simulink model "uz_mpc_6ph_sca"  (R2022b)
settings: Solver=FixedStepDiscrete  StartTime=0.0  StopTime=ST  RelTol=1e-3
InitFcn:
  | clear
  | clc
  | 
  | f_clock = 100e6;        % IP core clock freq in Hz
  | t_clock = 1/f_clock;    % IP core sample time in s
  | 
  | f_ADC =100e3;           % ADC interrupt freq in Hz
  | t_ADC = 1/f_ADC;        % ADC sample time in s
  | Ts = t_ADC;
  | 
  | % amplitude of sinusoidal signal sources
  | A = 0.1;
  | 
  | % machine parameters
  | Rs = 0.27;              % Phase resistance in Ohm
  | psi_pm = 0.19;          % PM flux linkage in Vs
  | Ld = 1.7e-3;            % d-inductance in H
  | Lq = 3.8e-3;            % q-inductance in H
  | Lx = 2.4e-3;            % x-inductance in H
  | Ly = 2.5e-3;            % y-inductance in H
  | p = 5;                  % pole pairs
  | 
  | VR = 400;               % Rated eff. line-line voltage in V
  | IR = 10/sqrt(2);             % Rated eff. phase current in A
  | % IR = 14.142;
  | nR = 3000;              % Rated mechanical speed in 1/min
  | 
  | % p.u. base units acc. to T.Geyer, Model predictive control of high power
  | % converters and industrial drives. Hoboken, NJ, USA: Wiley, 2016, Chapter 2.1.2
  | VB = sqrt(2/3)*VR;
  | IB = sqrt(2)*IR;
  | omegaB = nR*2*pi()/60*p;
  | ZB = VB/IB;
  | LB = ZB/omegaB;
  | SB = 3/2 *VB*IB;
  | psiB = VB/omegaB;
  | TB = psiB*IB;
  | 
  | %pre calculated constants - check results regarding fixd_type_constants!!!
  | Rs_over_ZB = Rs/ZB;
  | Ts_times_ZB_over_Ld = Ts*ZB/Ld;
  | Ts_times_ZB_over_Lq = Ts*ZB/Lq;
  | Ts_times_ZB_over_Lx = Ts*ZB/Lx;
  | Ts_times_ZB_over_Ly = Ts*ZB/Ly;
  | Ld_over_LB = Ld/LB;
  | Lq_over_LB = Lq/LB;
  | Ld_minus_Lq_over_LB = (Ld-Lq)/LB;
  | psi_pm_over_psiB = psi_pm/psiB;
  | 
  | % fixed-point data types
  | pu_fixdt_type = fixdt(1,18,15); % output data type of pu values
  | % fixdt_type_dq_currents = fixdt(1,27,16);
  | fixdt_type_dq_currents = fixdt(1,27,24);
  | fixdt_type_xy_currents = fixdt(1,18,11);
  | fixdt_type_dqxy_ref_currents = fixdt(1,18,15);
  | fixdt_type_dqxy_voltages = fixdt(1,27,24);
  | fixdt_type_angle = fixdt(1,24,20);
  | % fixdt_type_sin_cos = fixdt(1,18,16);
  | fixdt_type_sin_cos = fixdt(1,27,20);
  | fixdt_type_lambda = fixdt(0,18,17);
  | ... (+38 lines)
libraries: nesl_utility x44, fl_lib x41, simulink x23, ee_lib x12, hdlsllib x2, spsAlphaBetaZerotodq0Lib x1, batteryecm_lib x1
(part 3 of 4)

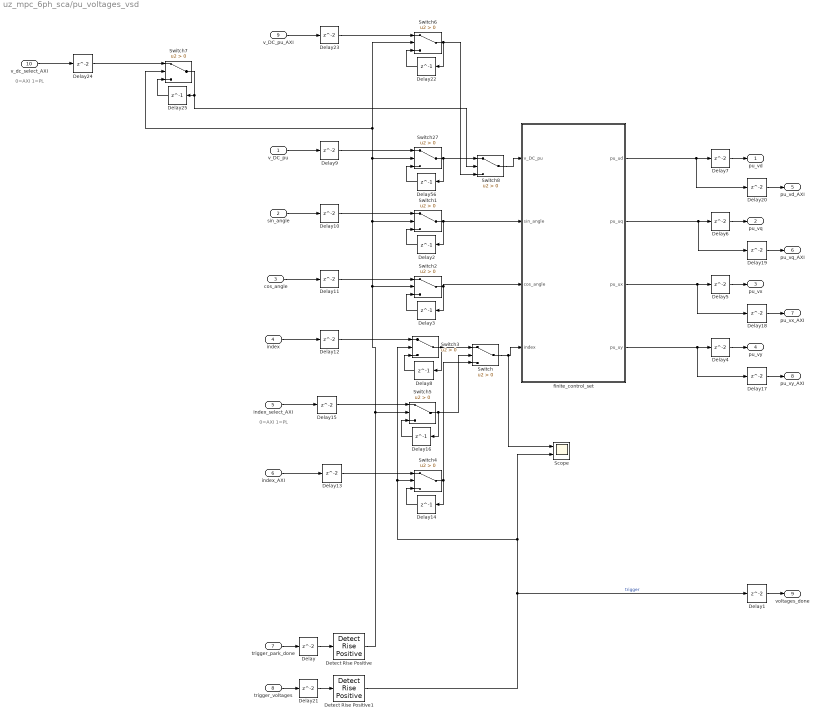
== system uz_mpc_6ph_sca/pu_voltages_vsd ==
  note: 0=AXI 1=PL
  note: 0=AXI 1=PL
  v_DC_pu : Inport  OutDataTypeStr=fixdt_type_constants
  sin_angle : Inport  Port=2  OutDataTypeStr=fixdt_type_sin_cos
  cos_angle : Inport  Port=3  OutDataTypeStr=fixdt_type_sin_cos
  index : Inport  Port=4
  index_select_AXI : Inport  Port=5
  index_AXI : Inport  Port=6
  trigger_park_done : Inport  Port=7
  trigger_voltages : Inport  Port=8
  v_DC_pu_AXI : Inport  Port=9  OutDataTypeStr=fixdt_type_constants
  v_dc_select_AXI : Inport  Port=10
  Delay{,1,4..7,9..11,17..21,23} (15 alike) : Delay
  Delay{12..13,15,24} (4 alike) : Delay  InitialCondition=1
  Delay{8,14,16,25} (4 alike) : Delay  DelayLength=1  InitialCondition=1
  Delay{2..3,22,56} (4 alike) : Delay  DelayLength=1
  Detect Rise Positive : simulink/Logic and Bit Operations/Detect Rise Positive  vinit=0  OutDataTypeStr=boolean
  Detect Rise Positive1 : simulink/Logic and Bit Operations/Detect Rise Positive  vinit=0  OutDataTypeStr=boolean
  Scope : Scope  NumInputPorts=2
  Switch : Switch  Criteria=u2 > Threshold  SaturateOnIntegerOverflow=off  InputSameDT=off
  Switch1 : Switch  Criteria=u2 > Threshold  OutDataTypeStr=fixdt_type_sin_cos  SaturateOnIntegerOverflow=off  InputSameDT=off
  Switch2 : Switch  Criteria=u2 > Threshold  OutDataTypeStr=fixdt_type_sin_cos  SaturateOnIntegerOverflow=off  InputSameDT=off
  Switch27 : Switch  Criteria=u2 > Threshold  OutDataTypeStr=fixdt_type_constants  SaturateOnIntegerOverflow=off  InputSameDT=off
  Switch{3..5,7} (4 alike) : Switch  Criteria=u2 > Threshold  OutDataTypeStr=fixdt_type_polepairs  SaturateOnIntegerOverflow=off  InputSameDT=off
  Switch6 : Switch  Criteria=u2 > Threshold  OutDataTypeStr=fixdt_type_constants  SaturateOnIntegerOverflow=off  InputSameDT=off
  Switch8 : Switch  Criteria=u2 > Threshold  SaturateOnIntegerOverflow=off  InputSameDT=off
  finite_control_set : MATLAB Function  TreatAsAtomicUnit=on
  pu_vd : Outport
  pu_vq : Outport  Port=2
  pu_vx : Outport  Port=3
  pu_vy : Outport  Port=4
  pu_vd_AXI : Outport  Port=5
  pu_vq_AXI : Outport  Port=6
  pu_vx_AXI : Outport  Port=7
  pu_vy_AXI : Outport  Port=8
  voltages_done : Outport  Port=9
  wires:
  finite_control_set/1(pu_ud) -> Delay20/1, Delay7/1
  finite_control_set/2(pu_uq) -> Delay19/1, Delay6/1
  finite_control_set/3(pu_ux) -> Delay18/1, Delay5/1
  finite_control_set/4(pu_uy) -> Delay17/1, Delay4/1
  trigger_park_done/1 -> Delay/1
  Delay/1 -> Detect Rise Positive/1
  Delay56/1 -> Switch27/3
  v_DC_pu/1 -> Delay9/1
  Switch27/1 -> Delay56/1, Switch8/1
  sin_angle/1 -> Delay10/1
  Delay2/1 -> Switch1/3
  Switch1/1 -> finite_control_set/2(sin_angle), Delay2/1
  cos_angle/1 -> Delay11/1
  Delay3/1 -> Switch2/3
  Switch2/1 -> finite_control_set/3(cos_angle), Delay3/1
  Delay4/1 -> pu_vy/1
  Delay5/1 -> pu_vx/1
  Delay6/1 -> pu_vq/1
  Delay7/1 -> pu_vd/1
  Switch3/1 -> Delay8/1, Switch/1
  index/1 -> Delay12/1
  Delay8/1 -> Switch3/3
  Delay9/1 -> Switch27/1
  Delay10/1 -> Switch1/1
  Delay11/1 -> Switch2/1
  Delay12/1 -> Switch3/1
  Delay14/1 -> Switch4/3
  index_AXI/1 -> Delay13/1
  Switch4/1 -> Switch/3, Delay14/1
  Delay13/1 -> Switch4/1
  Delay16/1 -> Switch5/3
  index_select_AXI/1 -> Delay15/1
  Switch5/1 -> Switch/2, Delay16/1
  Delay15/1 -> Switch5/1
  Delay17/1 -> pu_vy_AXI/1
  Delay19/1 -> pu_vq_AXI/1
  Delay20/1 -> pu_vd_AXI/1
  Delay18/1 -> pu_vx_AXI/1
  Detect Rise Positive1/1 -> Scope/2, Switch3/2, Switch4/2, Delay1/1  "trigger"
  Delay1/1 -> voltages_done/1
  trigger_voltages/1 -> Delay21/1
  Delay21/1 -> Detect Rise Positive1/1
  Switch/1 -> Scope/1, finite_control_set/4(index)
  Switch6/1 -> Switch8/3, Delay22/1
  Delay22/1 -> Switch6/3
  v_DC_pu_AXI/1 -> Delay23/1
  Delay23/1 -> Switch6/1
  v_dc_select_AXI/1 -> Delay24/1
  Delay25/1 -> Switch7/3
  Switch7/1 -> Switch8/2, Delay25/1
  Delay24/1 -> Switch7/1
  Detect Rise Positive/1 -> Switch5/2, Switch2/2, Switch7/2, Switch6/2, Switch27/2, Switch1/2
  Switch8/1 -> finite_control_set/1(v_DC_pu)

== system uz_mpc_6ph_sca/uz_current_limit ==
  ia1_SI : Inport
  ib1_SI : Inport  Port=2
  ic1_SI : Inport  Port=3
  ia2_SI : Inport  Port=4
  ib2_SI : Inport  Port=5
  ic2_SI : Inport  Port=6
  i_max_ampere_AXI : Inport  Port=7
  reset_violation_AXI : Inport  Port=8
  trigger : Inport  Port=9
  Abs{,1..5} (6 alike) : Abs  SaturateOnIntegerOverflow=off
  Delay{,2..16} (16 alike) : Delay  DelayLength=1
  Delay{1,17..18,31} (4 alike) : Delay  DelayLength=1  InitialCondition=0
  Detect Rise Positive : simulink/Logic and Bit Operations/Detect Rise Positive  vinit=0  OutDataTypeStr=boolean
  Detect Rise Positive1 : simulink/Logic and Bit Operations/Detect Rise Positive  vinit=0  OutDataTypeStr=boolean
  Detect Rise Positive2 : simulink/Logic and Bit Operations/Detect Rise Positive  vinit=0  OutDataTypeStr=boolean
  Mux1 : Mux  Inputs=6
  OR : Logic  Operator=OR  Inputs=6  IconShape=distinctive  AllPortsSameDT=off  OutDataTypeStr=boolean
  RS_flipflop : Subsystem
  Relational Operator{,1..5} (6 alike) : RelationalOperator  Operator=>  OutDataTypeStr=boolean  RndMeth=Simplest  InputSameDT=off
  Switch{1..7,31} (8 alike) : Switch  Criteria=u2 > Threshold  SaturateOnIntegerOverflow=off  InputSameDT=off
  Terminator : Terminator
  si_currents : Scope  NumInputPorts=2
  current_limit_violated : Outport  VectorParamsAs1DForOutWhenUnconnected=off
  current_limit_violated_AXI : Outport  Port=2  VectorParamsAs1DForOutWhenUnconnected=off
  done : Outport  Port=3  VectorParamsAs1DForOutWhenUnconnected=off
  wires:
  Abs/1 -> Relational Operator/1
  Abs1/1 -> Relational Operator1/1
  Abs2/1 -> Relational Operator2/1
  Abs3/1 -> Relational Operator3/1
  Abs4/1 -> Relational Operator4/1
  Abs5/1 -> Relational Operator5/1
  Switch31/1 -> Relational Operator5/2, Relational Operator4/2, Relational Operator3/2, Relational Operator2/2, Relational Operator1/2, Relational Operator/2, Delay31/1
  trigger/1 -> Delay/1
  Delay/1 -> Detect Rise Positive/1
  Delay31/1 -> Switch31/3
  i_max_ampere_AXI/1 -> Delay1/1
  Delay1/1 -> Switch31/1
  ia1_SI/1 -> Delay7/1
  ib1_SI/1 -> Delay6/1
  ic1_SI/1 -> Delay5/1
  ia2_SI/1 -> Delay4/1
  ib2_SI/1 -> Delay3/1
  ic2_SI/1 -> Delay2/1
  Delay7/1 -> Switch1/1
  Delay6/1 -> Switch2/1
  Delay5/1 -> Switch3/1
  Delay4/1 -> Switch4/1
  Delay3/1 -> Switch5/1
  Delay2/1 -> Switch6/1
  Detect Rise Positive/1 -> Switch7/2, Switch6/2, Switch5/2, Switch4/2, Switch3/2, Switch2/2, Switch1/2, Switch31/2, Delay16/1
  Delay11/1 -> Switch6/3
  Delay13/1 -> Switch5/3
  Delay12/1 -> Switch4/3
  Delay10/1 -> Switch3/3
  Delay9/1 -> Switch2/3
  Delay8/1 -> Switch1/3
  Switch1/1 -> Mux1/1, Abs/1, Delay8/1
  Switch2/1 -> Delay9/1, Mux1/2, Abs1/1
  Switch3/1 -> Delay10/1, Mux1/3, Abs2/1
  Switch4/1 -> Delay12/1, Mux1/4, Abs3/1
  Switch5/1 -> Delay13/1, Mux1/5, Abs4/1
  Switch6/1 -> Delay11/1, Mux1/6, Abs5/1
  Relational Operator/1 -> OR/1
  Relational Operator1/1 -> OR/2
  Relational Operator2/1 -> OR/3
  Relational Operator3/1 -> OR/4
  Relational Operator5/1 -> OR/6
  OR/1 -> Detect Rise Positive1/1
  Delay16/1 -> done/1
  Delay15/1 -> current_limit_violated_AXI/1
  Relational Operator4/1 -> OR/5
  Mux1/1 -> si_currents/1
  Delay14/1 -> si_currents/2, current_limit_violated/1
  RS_flipflop/1(Q) -> Delay15/1, Delay14/1
  RS_flipflop/2(!Q) -> Terminator/1
  reset_violation_AXI/1 -> Delay17/1
  Delay18/1 -> Switch7/3
  Switch7/1 -> Delay18/1, Detect Rise Positive2/1
  Delay17/1 -> Switch7/1
  Detect Rise Positive1/1 -> RS_flipflop/1(Set)
  Detect Rise Positive2/1 -> RS_flipflop/2(Reset)

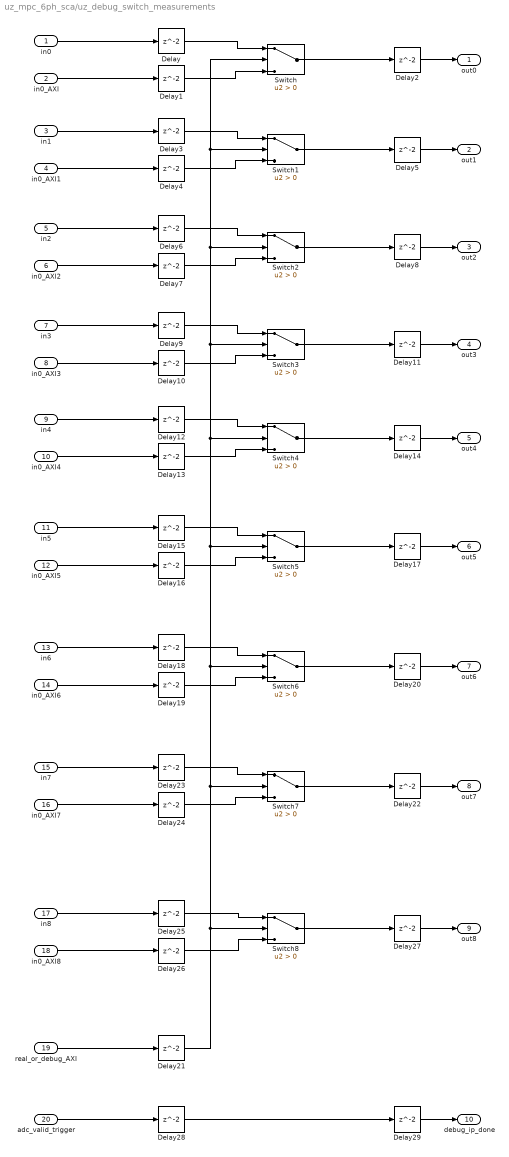
== system uz_mpc_6ph_sca/uz_debug_switch_measurements ==
  in0 : Inport
  in0_AXI : Inport  Port=2
  in1 : Inport  Port=3
  in0_AXI1 : Inport  Port=4
  in2 : Inport  Port=5
  in0_AXI2 : Inport  Port=6
  in3 : Inport  Port=7
  in0_AXI3 : Inport  Port=8
  in4 : Inport  Port=9
  in0_AXI4 : Inport  Port=10
  in5 : Inport  Port=11
  in0_AXI5 : Inport  Port=12
  in6 : Inport  Port=13
  in0_AXI6 : Inport  Port=14
  in7 : Inport  Port=15
  in0_AXI7 : Inport  Port=16
  in8 : Inport  Port=17
  in0_AXI8 : Inport  Port=18
  real_or_debug_AXI : Inport  Port=19
  adc_valid_trigger : Inport  Port=20
  Delay{,1..29} (30 alike) : Delay
  Switch{,1..8} (9 alike) : Switch  Criteria=u2 > Threshold  SaturateOnIntegerOverflow=off  InputSameDT=off
  out0 : Outport  VectorParamsAs1DForOutWhenUnconnected=off
  out1 : Outport  Port=2  VectorParamsAs1DForOutWhenUnconnected=off
  out2 : Outport  Port=3  VectorParamsAs1DForOutWhenUnconnected=off
  out3 : Outport  Port=4  VectorParamsAs1DForOutWhenUnconnected=off
  out4 : Outport  Port=5  VectorParamsAs1DForOutWhenUnconnected=off
  out5 : Outport  Port=6  VectorParamsAs1DForOutWhenUnconnected=off
  out6 : Outport  Port=7  VectorParamsAs1DForOutWhenUnconnected=off
  out7 : Outport  Port=8  VectorParamsAs1DForOutWhenUnconnected=off
  out8 : Outport  Port=9  VectorParamsAs1DForOutWhenUnconnected=off
  debug_ip_done : Outport  Port=10  VectorParamsAs1DForOutWhenUnconnected=off
  wires:
  in0/1 -> Delay/1
  in0_AXI/1 -> Delay1/1
  Delay/1 -> Switch/1
  Delay1/1 -> Switch/3
  Switch/1 -> Delay2/1
  Delay2/1 -> out0/1
  in0_AXI1/1 -> Delay4/1
  Delay5/1 -> out1/1
  in1/1 -> Delay3/1
  Delay4/1 -> Switch1/3
  Delay3/1 -> Switch1/1
  Switch1/1 -> Delay5/1
  in0_AXI2/1 -> Delay7/1
  Delay8/1 -> out2/1
  in2/1 -> Delay6/1
  Delay7/1 -> Switch2/3
  Delay6/1 -> Switch2/1
  Switch2/1 -> Delay8/1
  in0_AXI3/1 -> Delay10/1
  Delay11/1 -> out3/1
  in3/1 -> Delay9/1
  Delay10/1 -> Switch3/3
  Delay9/1 -> Switch3/1
  Switch3/1 -> Delay11/1
  in0_AXI4/1 -> Delay13/1
  Delay14/1 -> out4/1
  in4/1 -> Delay12/1
  Delay13/1 -> Switch4/3
  Delay12/1 -> Switch4/1
  Switch4/1 -> Delay14/1
  in0_AXI5/1 -> Delay16/1
  Delay17/1 -> out5/1
  in5/1 -> Delay15/1
  Delay16/1 -> Switch5/3
  Delay15/1 -> Switch5/1
  Switch5/1 -> Delay17/1
  in0_AXI6/1 -> Delay19/1
  Delay20/1 -> out6/1
  in6/1 -> Delay18/1
  Delay19/1 -> Switch6/3
  Delay18/1 -> Switch6/1
  Switch6/1 -> Delay20/1
  real_or_debug_AXI/1 -> Delay21/1
  Delay22/1 -> out7/1
  Delay23/1 -> Switch7/1
  Delay24/1 -> Switch7/3
  Switch7/1 -> Delay22/1
  in0_AXI7/1 -> Delay24/1
  in7/1 -> Delay23/1
  in0_AXI8/1 -> Delay26/1
  in8/1 -> Delay25/1
  Delay27/1 -> out8/1
  Switch8/1 -> Delay27/1
  Delay25/1 -> Switch8/1
  Delay26/1 -> Switch8/3
  Delay21/1 -> Switch/2, Switch1/2, Switch2/2, Switch3/2, Switch4/2, Switch5/2, Switch6/2, Switch7/2, Switch8/2
  Delay28/1 -> Delay29/1
  Delay29/1 -> debug_ip_done/1
  adc_valid_trigger/1 -> Delay28/1

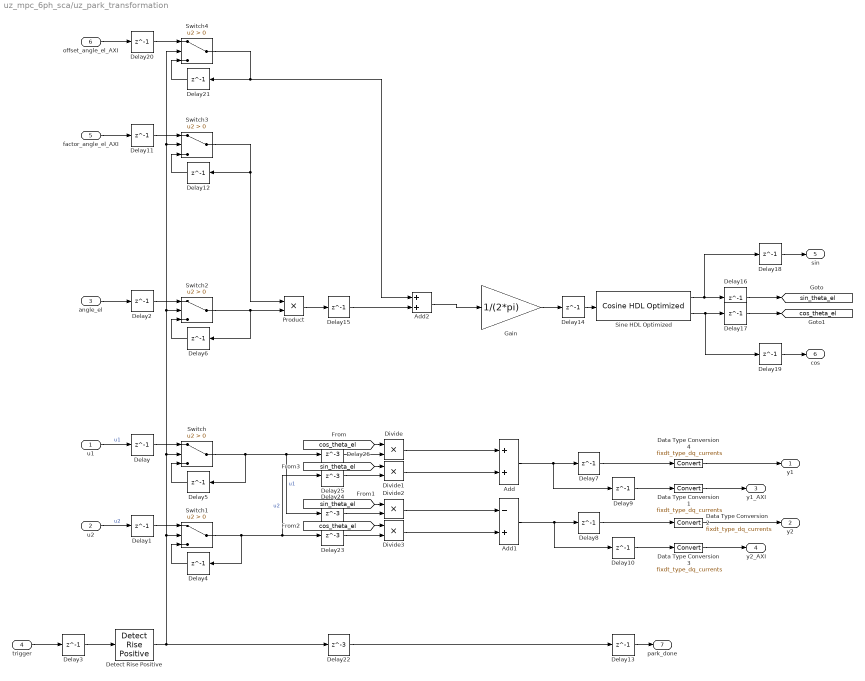
== system uz_mpc_6ph_sca/uz_park_transformation ==
  u1 : Inport
  u2 : Inport  Port=2
  angle_el : Inport  Port=3
  trigger : Inport  Port=4
  factor_angle_el_AXI : Inport  Port=5
  offset_angle_el_AXI : Inport  Port=6
  Add : Sum  OutDataTypeStr=fixdt(1,27,16)
  Add1 : Sum  Inputs=-+  OutDataTypeStr=fixdt(1,27,16)
  Add2 : Sum  AccumDataTypeStr=fixdt(1,27,20)
  Data Type Conversion{1..4} (4 alike) : DataTypeConversion  OutDataTypeStr=fixdt_type_dq_currents  SaturateOnIntegerOverflow=off  RndMeth=Floor
  Delay{,1..21} (22 alike) : Delay  DelayLength=1
  Delay{22..26} (5 alike) : Delay  DelayLength=3
  Detect Rise Positive : simulink/Logic and Bit Operations/Detect Rise Positive  vinit=0  OutDataTypeStr=boolean
  Divide{,1..3} (4 alike) : Product  Inputs=**  OutDataTypeStr=fixdt(1,27,16)
  Gain : Gain  Gain=1/(2*pi)  OutDataTypeStr=fixdt(1,27,20)
  Product : Product  OutDataTypeStr=fixdt(1,27,20)
  Sine HDL Optimized : hdlsllib/Lookup Tables/Cosine HDL Optimized  OutputFormula=sin(2*pi*u) and cos(2*pi*u)  NumDataPoints=256  TableDataTypeStr=fixdt(0,26,20)  SimulateLUTROMDelay=off
  Switch{,1..4} (5 alike) : Switch  Criteria=u2 > Threshold  SaturateOnIntegerOverflow=off  InputSameDT=off
  y1 : Outport  VectorParamsAs1DForOutWhenUnconnected=off
  y2 : Outport  Port=2  VectorParamsAs1DForOutWhenUnconnected=off
  y1_AXI : Outport  Port=3  VectorParamsAs1DForOutWhenUnconnected=off
  y2_AXI : Outport  Port=4  VectorParamsAs1DForOutWhenUnconnected=off
  sin : Outport  Port=5  VectorParamsAs1DForOutWhenUnconnected=off
  cos : Outport  Port=6  VectorParamsAs1DForOutWhenUnconnected=off
  park_done : Outport  Port=7  VectorParamsAs1DForOutWhenUnconnected=off
  tag scope: cos_theta_el=global, sin_theta_el=global
  wires:
  Switch1/1 -> Delay4/1, Delay25/1, Delay23/1  "u2"
  Divide2/1 -> Add1/1
  Divide3/1 -> Add1/2
  [cos_theta_el] -> Divide3/1
  Switch/1 -> Delay24/1, Delay26/1, Delay5/1  "u1"
  [sin_theta_el] -> Divide2/1
  Divide1/1 -> Add/2
  [cos_theta_el] -> Divide/1
  [sin_theta_el] -> Divide1/1
  Add/1 -> Delay9/1, Delay7/1
  Add1/1 -> Delay10/1, Delay8/1
  Divide/1 -> Add/1
  angle_el/1 -> Delay2/1
  Sine HDL Optimized/2 -> Delay19/1, Delay17/1
  Sine HDL Optimized/1 -> Delay18/1, Delay16/1
  Gain/1 -> Delay14/1
  u1/1 -> Delay/1  "u1"
  u2/1 -> Delay1/1  "u2"
  Delay/1 -> Switch/1
  Delay1/1 -> Switch1/1
  Delay2/1 -> Switch2/1
  trigger/1 -> Delay3/1
  Delay4/1 -> Switch1/3
  Delay5/1 -> Switch/3
  Delay6/1 -> Switch2/3
  Delay7/1 -> Data Type Conversion4/1
  Switch2/1 -> Product/2, Delay6/1
  Switch3/1 -> Product/1, Delay12/1
  factor_angle_el_AXI/1 -> Delay11/1
  Delay12/1 -> Switch3/3
  Delay11/1 -> Switch3/1
  Product/1 -> Delay15/1
  Delay3/1 -> Detect Rise Positive/1
  Delay13/1 -> park_done/1
  Delay14/1 -> Sine HDL Optimized/1
  Delay16/1 -> [sin_theta_el]
  Delay17/1 -> [cos_theta_el]
  Delay18/1 -> sin/1
  Delay19/1 -> cos/1
  Add2/1 -> Gain/1
  Delay20/1 -> Switch4/1
  Switch4/1 -> Add2/1, Delay21/1
  Detect Rise Positive/1 -> Delay22/1, Switch1/2, Switch/2, Switch4/2, Switch3/2, Switch2/2
  Delay21/1 -> Switch4/3
  offset_angle_el_AXI/1 -> Delay20/1
  Delay15/1 -> Add2/2
  Delay22/1 -> Delay13/1
  Delay23/1 -> Divide3/2
  Delay24/1 -> Divide2/2
  Delay25/1 -> Divide1/2
  Delay26/1 -> Divide/2
  Data Type Conversion4/1 -> y1/1
  Delay9/1 -> Data Type Conversion1/1
  Delay8/1 -> Data Type Conversion2/1
  Delay10/1 -> Data Type Conversion3/1
  Data Type Conversion1/1 -> y1_AXI/1
  Data Type Conversion2/1 -> y2/1
  Data Type Conversion3/1 -> y2_AXI/1

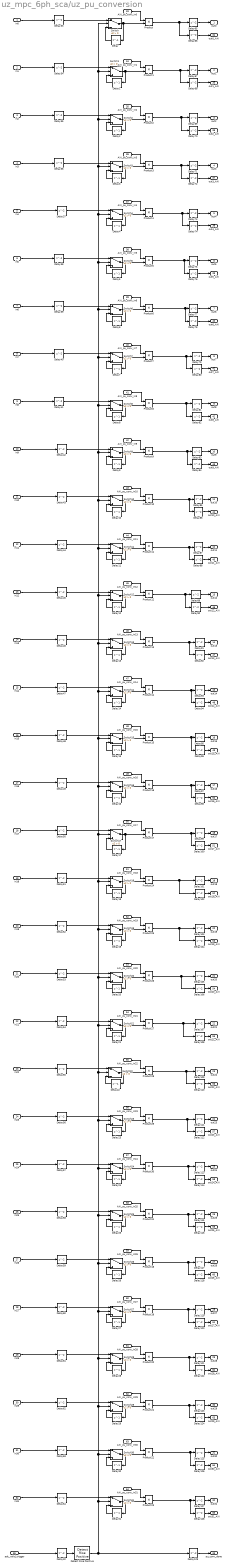
== system uz_mpc_6ph_sca/uz_pu_conversion ==
  in0 : Inport  OutDataTypeStr=fixdt(1,27,15)
  in1 : Inport  Port=2  OutDataTypeStr=fixdt(1,27,15)
  in2 : Inport  Port=3  OutDataTypeStr=fixdt(1,27,15)
  in3 : Inport  Port=4  OutDataTypeStr=fixdt(1,27,15)
  in4 : Inport  Port=5  OutDataTypeStr=fixdt(1,27,15)
  in5 : Inport  Port=6  OutDataTypeStr=fixdt(1,27,15)
  in6 : Inport  Port=7  OutDataTypeStr=fixdt(1,27,15)
  in7 : Inport  Port=8  OutDataTypeStr=fixdt(1,27,15)
  in8 : Inport  Port=9  OutDataTypeStr=fixdt(1,27,15)
  in9 : Inport  Port=10  OutDataTypeStr=fixdt(1,27,15)
  in10 : Inport  Port=11  OutDataTypeStr=fixdt(1,27,15)
  in11 : Inport  Port=12  OutDataTypeStr=fixdt(1,27,15)
  in12 : Inport  Port=13  OutDataTypeStr=fixdt(1,27,15)
  in13 : Inport  Port=14  OutDataTypeStr=fixdt(1,27,15)
  in14 : Inport  Port=15  OutDataTypeStr=fixdt(1,27,15)
  in15 : Inport  Port=16  OutDataTypeStr=fixdt(1,27,15)
  in16 : Inport  Port=17  OutDataTypeStr=fixdt(1,27,15)
  in17 : Inport  Port=18  OutDataTypeStr=fixdt(1,27,15)
  in18 : Inport  Port=19  OutDataTypeStr=fixdt(1,27,15)
  in19 : Inport  Port=20  OutDataTypeStr=fixdt(1,27,15)
  in20 : Inport  Port=21  OutDataTypeStr=fixdt(1,27,15)
  in21 : Inport  Port=22  OutDataTypeStr=fixdt(1,27,15)
  in22 : Inport  Port=23  OutDataTypeStr=fixdt(1,27,15)
  in23 : Inport  Port=24  OutDataTypeStr=fixdt(1,27,15)
  in24 : Inport  Port=25  OutDataTypeStr=fixdt(1,27,15)
  in25 : Inport  Port=26  OutDataTypeStr=fixdt(1,27,15)
  in26 : Inport  Port=27  OutDataTypeStr=fixdt(1,27,15)
  in27 : Inport  Port=28  OutDataTypeStr=fixdt(1,27,15)
  in28 : Inport  Port=29  OutDataTypeStr=fixdt(1,27,15)
  in29 : Inport  Port=30  OutDataTypeStr=fixdt(1,27,15)
  in30 : Inport  Port=31  OutDataTypeStr=fixdt(1,27,15)
  in31 : Inport  Port=32  OutDataTypeStr=fixdt(1,27,15)
  AXI_pu_conv_in0 : Inport  Port=33  OutDataTypeStr=fixdt(0,18,18)
  AXI_pu_conv_in1 : Inport  Port=34  OutDataTypeStr=fixdt(0,18,18)
  AXI_pu_conv_in2 : Inport  Port=35  OutDataTypeStr=fixdt(0,18,18)
  AXI_pu_conv_in3 : Inport  Port=36  OutDataTypeStr=fixdt(0,18,18)
  AXI_pu_conv_in4 : Inport  Port=37  OutDataTypeStr=fixdt(0,18,18)
  AXI_pu_conv_in5 : Inport  Port=38  OutDataTypeStr=fixdt(0,18,18)
  AXI_pu_conv_in6 : Inport  Port=39  OutDataTypeStr=fixdt(0,18,18)
  AXI_pu_conv_in7 : Inport  Port=40  OutDataTypeStr=fixdt(0,18,18)
  AXI_pu_conv_in8 : Inport  Port=41  OutDataTypeStr=fixdt(0,18,18)
  AXI_pu_conv_in9 : Inport  Port=42  OutDataTypeStr=fixdt(0,18,18)
  AXI_pu_conv_in10 : Inport  Port=43  OutDataTypeStr=fixdt(0,18,18)
  AXI_pu_conv_in11 : Inport  Port=44  OutDataTypeStr=fixdt(0,18,18)
  AXI_pu_conv_in12 : Inport  Port=45  OutDataTypeStr=fixdt(0,18,18)
  AXI_pu_conv_in13 : Inport  Port=46  OutDataTypeStr=fixdt(0,18,18)
  AXI_pu_conv_in14 : Inport  Port=47  OutDataTypeStr=fixdt(0,18,18)
  AXI_pu_conv_in15 : Inport  Port=48  OutDataTypeStr=fixdt(0,18,18)
  AXI_pu_conv_in16 : Inport  Port=49  OutDataTypeStr=fixdt(0,18,18)
  AXI_pu_conv_in17 : Inport  Port=50  OutDataTypeStr=fixdt(0,18,18)
  AXI_pu_conv_in18 : Inport  Port=51  OutDataTypeStr=fixdt(0,18,18)
  AXI_pu_conv_in19 : Inport  Port=52  OutDataTypeStr=fixdt(0,18,18)
  AXI_pu_conv_in20 : Inport  Port=53  OutDataTypeStr=fixdt(0,18,18)
  AXI_pu_conv_in21 : Inport  Port=54  OutDataTypeStr=fixdt(0,18,18)
  AXI_pu_conv_in22 : Inport  Port=55  OutDataTypeStr=fixdt(0,18,18)
  AXI_pu_conv_in23 : Inport  Port=56  OutDataTypeStr=fixdt(0,18,18)
  AXI_pu_conv_in24 : Inport  Port=57  OutDataTypeStr=fixdt(0,18,18)
  AXI_pu_conv_in25 : Inport  Port=58  OutDataTypeStr=fixdt(0,18,18)
  AXI_pu_conv_in26 : Inport  Port=59  OutDataTypeStr=fixdt(0,18,18)
  AXI_pu_conv_in27 : Inport  Port=60  OutDataTypeStr=fixdt(0,18,18)
  AXI_pu_conv_in28 : Inport  Port=61  OutDataTypeStr=fixdt(0,18,18)
  AXI_pu_conv_in29 : Inport  Port=62  OutDataTypeStr=fixdt(0,18,18)
  AXI_pu_conv_in30 : Inport  Port=63  OutDataTypeStr=fixdt(0,18,18)
  AXI_pu_conv_in31 : Inport  Port=64  OutDataTypeStr=fixdt(0,18,18)
  adc_valid_trigger : Inport  Port=65  OutDataTypeStr=boolean
  Delay{,1..31} (32 alike) : Delay  DelayLength=1
  Delay{32..129} (98 alike) : Delay
  Detect Rise Positive : simulink/Logic and Bit Operations/Detect Rise Positive  vinit=0  OutDataTypeStr=boolean
  Product{,1..31} (32 alike) : Product  OutDataTypeStr=pu_fixdt_type
  Switch{,1..31} (32 alike) : Switch  Criteria=u2 > Threshold  SaturateOnIntegerOverflow=off  InputSameDT=off
  out0 : Outport
  out1 : Outport  Port=2
  out2 : Outport  Port=3
  out3 : Outport  Port=4
  out4 : Outport  Port=5
  out5 : Outport  Port=6
  out6 : Outport  Port=7
  out7 : Outport  Port=8
  out8 : Outport  Port=9
  out9 : Outport  Port=10
  out10 : Outport  Port=11
  out11 : Outport  Port=12
  out12 : Outport  Port=13
  out13 : Outport  Port=14
  out14 : Outport  Port=15
  out15 : Outport  Port=16
  out16 : Outport  Port=17
  out17 : Outport  Port=18
  out18 : Outport  Port=19
  out19 : Outport  Port=20
  out20 : Outport  Port=21
  out21 : Outport  Port=22
  out22 : Outport  Port=23
  out23 : Outport  Port=24
  out24 : Outport  Port=25
  out25 : Outport  Port=26
  out26 : Outport  Port=27
  out27 : Outport  Port=28
  out28 : Outport  Port=29
  out29 : Outport  Port=30
  out30 : Outport  Port=31
  out31 : Outport  Port=32
  pu_conv_done : Outport  Port=33  OutDataTypeStr=boolean  LockScale=on
  out0_AXI : Outport  Port=34
  out1_AXI : Outport  Port=35
  out2_AXI : Outport  Port=36
  out3_AXI : Outport  Port=37
  out4_AXI : Outport  Port=38
  out5_AXI : Outport  Port=39
  out6_AXI : Outport  Port=40
  out7_AXI : Outport  Port=41
  out8_AXI : Outport  Port=42
  out9_AXI : Outport  Port=43
  out10_AXI : Outport  Port=44
  out11_AXI : Outport  Port=45
  out12_AXI : Outport  Port=46
  out13_AXI : Outport  Port=47
  out14_AXI : Outport  Port=48
  out15_AXI : Outport  Port=49
  out16_AXI : Outport  Port=50
  out17_AXI : Outport  Port=51
  out18_AXI : Outport  Port=52
  out19_AXI : Outport  Port=53
  out20_AXI : Outport  Port=54
  out21_AXI : Outport  Port=55
  out22_AXI : Outport  Port=56
  out23_AXI : Outport  Port=57
  out24_AXI : Outport  Port=58
  out25_AXI : Outport  Port=59
  out26_AXI : Outport  Port=60
  out27_AXI : Outport  Port=61
  out28_AXI : Outport  Port=62
  out29_AXI : Outport  Port=63
  out30_AXI : Outport  Port=64
  out31_AXI : Outport  Port=65
  wires:
  AXI_pu_conv_in0/1 -> Product/1
  Product/1 -> Delay65/1, Delay66/1
  AXI_pu_conv_in1/1 -> Product1/1
  Product1/1 -> Delay67/1, Delay68/1
  AXI_pu_conv_in2/1 -> Product2/1
  Product3/1 -> Delay71/1, Delay72/1
  Product2/1 -> Delay69/1, Delay70/1
  AXI_pu_conv_in3/1 -> Product3/1
  AXI_pu_conv_in4/1 -> Product4/1
  AXI_pu_conv_in7/1 -> Product7/1
  Product7/1 -> Delay79/1, Delay80/1
  Product6/1 -> Delay77/1, Delay78/1
  Product5/1 -> Delay75/1, Delay76/1
  AXI_pu_conv_in6/1 -> Product6/1
  Product4/1 -> Delay73/1, Delay74/1
  AXI_pu_conv_in5/1 -> Product5/1
  AXI_pu_conv_in8/1 -> Product8/1
  AXI_pu_conv_in11/1 -> Product11/1
  Product10/1 -> Delay85/1, Delay86/1
  Product11/1 -> Delay87/1, Delay88/1
  AXI_pu_conv_in10/1 -> Product10/1
  AXI_pu_conv_in9/1 -> Product9/1
  AXI_pu_conv_in14/1 -> Product14/1
  Product12/1 -> Delay89/1, Delay90/1
  AXI_pu_conv_in13/1 -> Product13/1
  AXI_pu_conv_in15/1 -> Product15/1
  Product9/1 -> Delay83/1, Delay84/1
  Product14/1 -> Delay93/1, Delay94/1
  Product13/1 -> Delay91/1, Delay92/1
  Product8/1 -> Delay81/1, Delay82/1
  AXI_pu_conv_in12/1 -> Product12/1
  Product15/1 -> Delay95/1, Delay96/1
  Product30/1 -> Delay113/1, Delay114/1
  Product23/1 -> Delay127/1, Delay128/1
  AXI_pu_conv_in28/1 -> Product20/1
  AXI_pu_conv_in29/1 -> Product21/1
  Product20/1 -> Delay121/1, Delay122/1
  Product31/1 -> Delay115/1, Delay116/1
  AXI_pu_conv_in25/1 -> Product31/1
  AXI_pu_conv_in24/1 -> Product30/1
  Product18/1 -> Delay117/1, Delay118/1
  AXI_pu_conv_in27/1 -> Product19/1
  Product19/1 -> Delay119/1, Delay120/1
  AXI_pu_conv_in31/1 -> Product23/1
  AXI_pu_conv_in16/1 -> Product16/1
  AXI_pu_conv_in26/1 -> Product18/1
  AXI_pu_conv_in19/1 -> Product25/1
  Product24/1 -> Delay101/1, Delay102/1
  Product25/1 -> Delay103/1, Delay104/1
  AXI_pu_conv_in18/1 -> Product24/1
  AXI_pu_conv_in17/1 -> Product17/1
  AXI_pu_conv_in22/1 -> Product28/1
  AXI_pu_conv_in30/1 -> Product22/1
  Product26/1 -> Delay105/1, Delay106/1
  AXI_pu_conv_in21/1 -> Product27/1
  AXI_pu_conv_in23/1 -> Product29/1
  Product17/1 -> Delay99/1, Delay100/1
  Product28/1 -> Delay109/1, Delay110/1
  Product27/1 -> Delay107/1, Delay108/1
  Product21/1 -> Delay123/1, Delay124/1
  Product16/1 -> Delay97/1, Delay98/1
  AXI_pu_conv_in20/1 -> Product26/1
  Product29/1 -> Delay111/1, Delay112/1
  Switch/1 -> Product/2, Delay/1
  Delay/1 -> Switch/3
  Switch1/1 -> Product1/2, Delay1/1
  Delay1/1 -> Switch1/3
  Switch2/1 -> Product2/2, Delay2/1
  Delay2/1 -> Switch2/3
  Switch3/1 -> Product3/2, Delay3/1
  Delay3/1 -> Switch3/3
  Switch4/1 -> Product4/2, Delay4/1
  Delay4/1 -> Switch4/3
  Switch5/1 -> Product5/2, Delay5/1
  Delay5/1 -> Switch5/3
  Switch6/1 -> Product6/2, Delay6/1
  Delay6/1 -> Switch6/3
  Switch7/1 -> Product7/2, Delay7/1
  Delay7/1 -> Switch7/3
  Switch8/1 -> Product8/2, Delay8/1
  Delay8/1 -> Switch8/3
  Switch9/1 -> Product9/2, Delay9/1
  Delay9/1 -> Switch9/3
  Switch10/1 -> Product10/2, Delay10/1
  Delay10/1 -> Switch10/3
  Switch11/1 -> Product11/2, Delay11/1
  Delay11/1 -> Switch11/3
  Switch12/1 -> Product12/2, Delay12/1
  Delay12/1 -> Switch12/3
  Switch13/1 -> Product13/2, Delay13/1
  Delay13/1 -> Switch13/3
  Switch14/1 -> Product14/2, Delay14/1
  Delay14/1 -> Switch14/3
  Switch15/1 -> Product15/2, Delay15/1
  Delay15/1 -> Switch15/3
  Switch16/1 -> Product16/2, Delay16/1
  Delay16/1 -> Switch16/3
  Switch17/1 -> Product17/2, Delay17/1
  Delay17/1 -> Switch17/3
  Switch18/1 -> Product24/2, Delay18/1
  Delay18/1 -> Switch18/3
  Switch19/1 -> Product25/2, Delay19/1
  Delay19/1 -> Switch19/3
  Switch20/1 -> Product26/2, Delay20/1
  Delay20/1 -> Switch20/3
  Switch21/1 -> Product27/2, Delay21/1
  Delay21/1 -> Switch21/3
  Switch22/1 -> Product28/2, Delay22/1
  Delay22/1 -> Switch22/3
  Switch23/1 -> Product29/2, Delay23/1
  Delay23/1 -> Switch23/3
  Switch24/1 -> Product30/2, Delay24/1
  Delay24/1 -> Switch24/3
  Switch25/1 -> Product31/2, Delay25/1
  Delay25/1 -> Switch25/3
  Switch26/1 -> Product18/2, Delay26/1
  Delay26/1 -> Switch26/3
  Switch27/1 -> Product19/2, Delay27/1
  Delay27/1 -> Switch27/3
  Switch28/1 -> Product20/2, Delay28/1
  Delay28/1 -> Switch28/3
  Switch29/1 -> Product21/2, Delay29/1
  Delay29/1 -> Switch29/3
  Switch30/1 -> Product22/2, Delay30/1
  Delay30/1 -> Switch30/3
  Switch31/1 -> Product23/2, Delay31/1
  Delay31/1 -> Switch31/3
  Detect Rise Positive/1 -> Delay129/1, Switch31/2, Switch30/2, Switch29/2, Switch28/2, Switch27/2, Switch26/2, Switch25/2, Switch24/2, Switch23/2, Switch22/2, Switch21/2, Switch20/2, Switch19/2, Switch18/2, Switch17/2, Switch16/2, Switch15/2, Switch14/2, Switch13/2, Switch11/2, Switch10/2, Switch9/2, Switch7/2, Switch6/2, Switch5/2, Switch3/2, Switch2/2, Switch1/2, Switch/2, Switch4/2, Switch8/2, Switch12/2
  adc_valid_trigger/1 -> Delay32/1
  Product22/1 -> Delay125/1, Delay126/1
  Delay32/1 -> Detect Rise Positive/1
  in0/1 -> Delay33/1
  Delay33/1 -> Switch/1
  in1/1 -> Delay34/1
  Delay34/1 -> Switch1/1
  in2/1 -> Delay35/1
  Delay35/1 -> Switch2/1
  in3/1 -> Delay36/1
  Delay36/1 -> Switch3/1
  in4/1 -> Delay37/1
  Delay37/1 -> Switch4/1
  in5/1 -> Delay38/1
  Delay38/1 -> Switch5/1
  in6/1 -> Delay39/1
  Delay39/1 -> Switch6/1
  in7/1 -> Delay40/1
  Delay40/1 -> Switch7/1
  in8/1 -> Delay41/1
  Delay41/1 -> Switch8/1
  in9/1 -> Delay42/1
  Delay42/1 -> Switch9/1
  in10/1 -> Delay43/1
  Delay43/1 -> Switch10/1
  in11/1 -> Delay44/1
  Delay44/1 -> Switch11/1
  in12/1 -> Delay45/1
  Delay45/1 -> Switch12/1
  in13/1 -> Delay46/1
  Delay46/1 -> Switch13/1
  in14/1 -> Delay47/1
  Delay47/1 -> Switch14/1
  in15/1 -> Delay48/1
  Delay48/1 -> Switch15/1
  in16/1 -> Delay49/1
  Delay49/1 -> Switch16/1
  in17/1 -> Delay50/1
  Delay50/1 -> Switch17/1
  in18/1 -> Delay51/1
  Delay51/1 -> Switch18/1
  in19/1 -> Delay52/1
  Delay52/1 -> Switch19/1
  in20/1 -> Delay53/1
  Delay53/1 -> Switch20/1
  in21/1 -> Delay54/1
  Delay54/1 -> Switch21/1
  in22/1 -> Delay55/1
  Delay55/1 -> Switch22/1
  in23/1 -> Delay56/1
  Delay56/1 -> Switch23/1
  in24/1 -> Delay57/1
  Delay57/1 -> Switch24/1
  in25/1 -> Delay58/1
  Delay58/1 -> Switch25/1
  in26/1 -> Delay59/1
  Delay59/1 -> Switch26/1
  in27/1 -> Delay60/1
  Delay60/1 -> Switch27/1
  in28/1 -> Delay61/1
  Delay61/1 -> Switch28/1
  in29/1 -> Delay62/1
  Delay62/1 -> Switch29/1
  in30/1 -> Delay63/1
  Delay63/1 -> Switch30/1
  in31/1 -> Delay64/1
  Delay64/1 -> Switch31/1
  Delay65/1 -> out0/1
  Delay66/1 -> out0_AXI/1
  Delay67/1 -> out1/1
  Delay68/1 -> out1_AXI/1
  Delay69/1 -> out2/1
  Delay70/1 -> out2_AXI/1
  Delay71/1 -> out3/1
  Delay72/1 -> out3_AXI/1
  Delay73/1 -> out4/1
  Delay74/1 -> out4_AXI/1
  Delay75/1 -> out5/1
  Delay76/1 -> out5_AXI/1
  Delay77/1 -> out6/1
  Delay78/1 -> out6_AXI/1
  Delay79/1 -> out7/1
  Delay80/1 -> out7_AXI/1
  Delay81/1 -> out8/1
  Delay82/1 -> out8_AXI/1
  Delay83/1 -> out9/1
  Delay84/1 -> out9_AXI/1
  Delay85/1 -> out10/1
  Delay86/1 -> out10_AXI/1
  Delay87/1 -> out11/1
  Delay88/1 -> out11_AXI/1
  Delay89/1 -> out12/1
  Delay90/1 -> out12_AXI/1
  Delay91/1 -> out13/1
  Delay92/1 -> out13_AXI/1
  Delay93/1 -> out14/1
  Delay94/1 -> out14_AXI/1
  Delay95/1 -> out15/1
  Delay96/1 -> out15_AXI/1
  Delay97/1 -> out16/1
  Delay98/1 -> out16_AXI/1
  Delay99/1 -> out17/1
  Delay100/1 -> out17_AXI/1
  Delay101/1 -> out18/1
  Delay102/1 -> out18_AXI/1
  Delay103/1 -> out19/1
  Delay104/1 -> out19_AXI/1
  Delay105/1 -> out20/1
  Delay106/1 -> out20_AXI/1
  Delay107/1 -> out21/1
  Delay108/1 -> out21_AXI/1
  Delay109/1 -> out22/1
  Delay110/1 -> out22_AXI/1
  Delay111/1 -> out23/1
  Delay112/1 -> out23_AXI/1
  Delay113/1 -> out24/1
  Delay114/1 -> out24_AXI/1
  Delay115/1 -> out25/1
  Delay116/1 -> out25_AXI/1
  Delay117/1 -> out26/1
  Delay118/1 -> out26_AXI/1
  Delay119/1 -> out27/1
  Delay120/1 -> out27_AXI/1
  Delay121/1 -> out28/1
  Delay122/1 -> out28_AXI/1
  Delay123/1 -> out29/1
  Delay124/1 -> out29_AXI/1
  Delay125/1 -> out30/1
  Delay126/1 -> out30_AXI/1
  Delay127/1 -> out31/1
  Delay128/1 -> out31_AXI/1
  Delay129/1 -> pu_conv_done/1

== system uz_mpc_6ph_sca/uz_vsd_6ph_30deg ==
  a1 : Inport
  b1 : Inport  Port=2
  c1 : Inport  Port=3
  a2 : Inport  Port=4
  b2 : Inport  Port=5
  c2 : Inport  Port=6
  pu_conv_valid : Inport  Port=7
  Delay{,1..5} (6 alike) : Delay  DelayLength=1
  Delay{6..25} (20 alike) : Delay
  Detect Rise Positive : simulink/Logic and Bit Operations/Detect Rise Positive  vinit=0  OutDataTypeStr=boolean
  Switch{,1..5} (6 alike) : Switch  Criteria=u2 > Threshold  OutDataTypeStr=fixdt_type_vsd  SaturateOnIntegerOverflow=off  InputSameDT=off
  VSD_6ph_30deg : MATLAB Function  TreatAsAtomicUnit=on
  alpha : Outport  OutDataTypeStr=fixdt(1,18,11)  VectorParamsAs1DForOutWhenUnconnected=off
  beta : Outport  Port=2  OutDataTypeStr=fixdt(1,18,11)  VectorParamsAs1DForOutWhenUnconnected=off
  x1 : Outport  Port=3  OutDataTypeStr=fixdt(1,18,11)  VectorParamsAs1DForOutWhenUnconnected=off
  y1 : Outport  Port=4  OutDataTypeStr=fixdt(1,18,11)  VectorParamsAs1DForOutWhenUnconnected=off
  z1 : Outport  Port=5  OutDataTypeStr=fixdt(1,18,11)  VectorParamsAs1DForOutWhenUnconnected=off
  z2 : Outport  Port=6  OutDataTypeStr=fixdt(1,18,11)  VectorParamsAs1DForOutWhenUnconnected=off
  vsd_done : Outport  Port=7  VectorParamsAs1DForOutWhenUnconnected=off
  alpha_AXI : Outport  Port=8  OutDataTypeStr=fixdt(1,18,11)  VectorParamsAs1DForOutWhenUnconnected=off
  beta_AXI : Outport  Port=9  OutDataTypeStr=fixdt(1,18,11)  VectorParamsAs1DForOutWhenUnconnected=off
  x_AXI : Outport  Port=10  OutDataTypeStr=fixdt(1,18,11)  VectorParamsAs1DForOutWhenUnconnected=off
  y_AXI : Outport  Port=11  OutDataTypeStr=fixdt(1,18,11)  VectorParamsAs1DForOutWhenUnconnected=off
  z1_AXI : Outport  Port=12  OutDataTypeStr=fixdt(1,18,11)  VectorParamsAs1DForOutWhenUnconnected=off
  z2_AXI : Outport  Port=13  OutDataTypeStr=fixdt(1,18,11)  VectorParamsAs1DForOutWhenUnconnected=off
  wires:
  VSD_6ph_30deg/1(alpha) -> Delay20/1, Delay14/1
  VSD_6ph_30deg/2(beta) -> Delay21/1, Delay15/1
  VSD_6ph_30deg/3(x1) -> Delay22/1, Delay16/1
  VSD_6ph_30deg/4(y1) -> Delay23/1, Delay17/1
  VSD_6ph_30deg/5(z1) -> Delay24/1, Delay18/1
  VSD_6ph_30deg/6(z2) -> Delay25/1, Delay19/1
  pu_conv_valid/1 -> Delay6/1
  Detect Rise Positive/1 -> Switch5/2, Switch4/2, Switch3/2, Switch2/2, Switch1/2, Switch/2, Delay13/1
  Delay/1 -> Switch/3
  Switch/1 -> VSD_6ph_30deg/1(a1), Delay/1
  Delay1/1 -> Switch1/3
  Switch1/1 -> VSD_6ph_30deg/2(b1), Delay1/1
  Delay2/1 -> Switch2/3
  Switch2/1 -> VSD_6ph_30deg/3(c1), Delay2/1
  Delay3/1 -> Switch3/3
  Switch3/1 -> VSD_6ph_30deg/4(a2), Delay3/1
  Delay4/1 -> Switch4/3
  Switch4/1 -> VSD_6ph_30deg/5(b2), Delay4/1
  Delay5/1 -> Switch5/3
  Switch5/1 -> VSD_6ph_30deg/6(c2), Delay5/1
  a1/1 -> Delay7/1
  b1/1 -> Delay8/1
  c1/1 -> Delay9/1
  a2/1 -> Delay10/1
  b2/1 -> Delay11/1
  c2/1 -> Delay12/1
  Delay6/1 -> Detect Rise Positive/1
  Delay7/1 -> Switch/1
  Delay8/1 -> Switch1/1
  Delay9/1 -> Switch2/1
  Delay10/1 -> Switch3/1
  Delay11/1 -> Switch4/1
  Delay12/1 -> Switch5/1
  Delay13/1 -> vsd_done/1
  Delay14/1 -> alpha/1
  Delay15/1 -> beta/1
  Delay16/1 -> x1/1
  Delay17/1 -> y1/1
  Delay18/1 -> z1/1
  Delay19/1 -> z2/1
  Delay20/1 -> alpha_AXI/1
  Delay21/1 -> beta_AXI/1
  Delay22/1 -> x_AXI/1
  Delay23/1 -> y_AXI/1
  Delay24/1 -> z1_AXI/1
  Delay25/1 -> z2_AXI/1

== system uz_mpc_6ph_sca/ctrl_state_machine/Subsystem ==
  Set : Inport
  Reset : Inport  Port=2
  Constant1 : Constant  Value=0  OutDataTypeStr=uint32  SampleTime=-1
  Data Type Conversion1 : DataTypeConversion  OutDataTypeStr=boolean  SaturateOnIntegerOverflow=off  RndMeth=Floor
  Data Type Conversion2 : DataTypeConversion  OutDataTypeStr=boolean  SaturateOnIntegerOverflow=off  RndMeth=Floor
  Logical Operator : Logic  Operator=NOT  AllPortsSameDT=off  OutDataTypeStr=boolean
  Logical Operator1 : Logic  AllPortsSameDT=off  OutDataTypeStr=boolean
  Logical Operator2 : Logic  Operator=OR  AllPortsSameDT=off  OutDataTypeStr=boolean
  Logical Operator3 : Logic  Operator=NOT  AllPortsSameDT=off  OutDataTypeStr=boolean
  Logical Operator4 : Logic  Operator=OR  AllPortsSameDT=off  OutDataTypeStr=boolean
  Logical Operator5 : Logic  AllPortsSameDT=off  OutDataTypeStr=boolean
  Switch1 : Switch  Criteria=u2 > Threshold  Threshold=1  SaturateOnIntegerOverflow=off  InputSameDT=off
  Unit Delay : UnitDelay  InitialCondition=1  SampleTime=t_clock  HasFrameUpgradeWarning=on
  Q : Outport  VectorParamsAs1DForOutWhenUnconnected=off
  !Q : Outport  Port=2  VectorParamsAs1DForOutWhenUnconnected=off
  wires:
  Logical Operator/1 -> Logical Operator1/2, Logical Operator5/1
  Reset/1 -> Data Type Conversion2/1
  Constant1/1 -> Switch1/2
  Logical Operator4/1 -> Switch1/1
  Data Type Conversion1/1 -> Logical Operator2/1, Logical Operator4/1
  Switch1/1 -> Q/1, Unit Delay/1, Logical Operator3/1
  Logical Operator3/1 -> !Q/1
  Set/1 -> Data Type Conversion1/1
  Logical Operator2/1 -> Logical Operator1/1
  Unit Delay/1 -> Logical Operator2/2, Logical Operator5/2
  Logical Operator5/1 -> Logical Operator4/2
  Logical Operator1/1 -> Switch1/3
  Data Type Conversion2/1 -> Logical Operator/1

== system uz_mpc_6ph_sca/ctrl_state_machine/Subsystem2 ==
  Set : Inport
  Reset : Inport  Port=2
  Constant1 : Constant  Value=0  OutDataTypeStr=uint32  SampleTime=-1
  Data Type Conversion1 : DataTypeConversion  OutDataTypeStr=boolean  SaturateOnIntegerOverflow=off  RndMeth=Floor
  Data Type Conversion2 : DataTypeConversion  OutDataTypeStr=boolean  SaturateOnIntegerOverflow=off  RndMeth=Floor
  Logical Operator : Logic  Operator=NOT  AllPortsSameDT=off  OutDataTypeStr=boolean
  Logical Operator1 : Logic  AllPortsSameDT=off  OutDataTypeStr=boolean
  Logical Operator2 : Logic  Operator=OR  AllPortsSameDT=off  OutDataTypeStr=boolean
  Logical Operator3 : Logic  Operator=NOT  AllPortsSameDT=off  OutDataTypeStr=boolean
  Logical Operator4 : Logic  Operator=OR  AllPortsSameDT=off  OutDataTypeStr=boolean
  Logical Operator5 : Logic  AllPortsSameDT=off  OutDataTypeStr=boolean
  Switch1 : Switch  Criteria=u2 > Threshold  Threshold=1  SaturateOnIntegerOverflow=off  InputSameDT=off
  Unit Delay : UnitDelay  SampleTime=t_clock  HasFrameUpgradeWarning=on
  Q : Outport  VectorParamsAs1DForOutWhenUnconnected=off
  !Q : Outport  Port=2  VectorParamsAs1DForOutWhenUnconnected=off
  wires:
  Logical Operator/1 -> Logical Operator1/2, Logical Operator5/1
  Reset/1 -> Data Type Conversion2/1
  Constant1/1 -> Switch1/2
  Logical Operator4/1 -> Switch1/1
  Data Type Conversion1/1 -> Logical Operator2/1, Logical Operator4/1
  Switch1/1 -> Q/1, Unit Delay/1, Logical Operator3/1
  Logical Operator3/1 -> !Q/1
  Set/1 -> Data Type Conversion1/1
  Logical Operator2/1 -> Logical Operator1/1
  Unit Delay/1 -> Logical Operator2/2, Logical Operator5/2
  Logical Operator5/1 -> Logical Operator4/2
  Logical Operator1/1 -> Switch1/3
  Data Type Conversion2/1 -> Logical Operator/1

== system uz_mpc_6ph_sca/ctrl_state_machine/Subsystem4 ==
  Set : Inport
  Reset : Inport  Port=2
  Constant1 : Constant  Value=0  OutDataTypeStr=uint32  SampleTime=-1
  Data Type Conversion1 : DataTypeConversion  OutDataTypeStr=boolean  SaturateOnIntegerOverflow=off  RndMeth=Floor
  Data Type Conversion2 : DataTypeConversion  OutDataTypeStr=boolean  SaturateOnIntegerOverflow=off  RndMeth=Floor
  Logical Operator : Logic  Operator=NOT  AllPortsSameDT=off  OutDataTypeStr=boolean
  Logical Operator1 : Logic  AllPortsSameDT=off  OutDataTypeStr=boolean
  Logical Operator2 : Logic  Operator=OR  AllPortsSameDT=off  OutDataTypeStr=boolean
  Logical Operator3 : Logic  Operator=NOT  AllPortsSameDT=off  OutDataTypeStr=boolean
  Logical Operator4 : Logic  Operator=OR  AllPortsSameDT=off  OutDataTypeStr=boolean
  Logical Operator5 : Logic  AllPortsSameDT=off  OutDataTypeStr=boolean
  Switch1 : Switch  Criteria=u2 > Threshold  Threshold=1  SaturateOnIntegerOverflow=off  InputSameDT=off
  Unit Delay : UnitDelay  SampleTime=t_clock  HasFrameUpgradeWarning=on
  Q : Outport  VectorParamsAs1DForOutWhenUnconnected=off
  !Q : Outport  Port=2  VectorParamsAs1DForOutWhenUnconnected=off
  wires:
  Logical Operator/1 -> Logical Operator1/2, Logical Operator5/1
  Reset/1 -> Data Type Conversion2/1
  Constant1/1 -> Switch1/2
  Logical Operator4/1 -> Switch1/1
  Data Type Conversion1/1 -> Logical Operator2/1, Logical Operator4/1
  Switch1/1 -> Q/1, Unit Delay/1, Logical Operator3/1
  Logical Operator3/1 -> !Q/1
  Set/1 -> Data Type Conversion1/1
  Logical Operator2/1 -> Logical Operator1/1
  Unit Delay/1 -> Logical Operator2/2, Logical Operator5/2
  Logical Operator5/1 -> Logical Operator4/2
  Logical Operator1/1 -> Switch1/3
  Data Type Conversion2/1 -> Logical Operator/1

== system uz_mpc_6ph_sca/ctrl_state_machine/Subsystem7 ==
  Set : Inport
  Reset : Inport  Port=2
  Constant1 : Constant  Value=0  OutDataTypeStr=uint32  SampleTime=-1
  Data Type Conversion1 : DataTypeConversion  OutDataTypeStr=boolean  SaturateOnIntegerOverflow=off  RndMeth=Floor
  Data Type Conversion2 : DataTypeConversion  OutDataTypeStr=boolean  SaturateOnIntegerOverflow=off  RndMeth=Floor
  Logical Operator : Logic  Operator=NOT  AllPortsSameDT=off  OutDataTypeStr=boolean
  Logical Operator1 : Logic  AllPortsSameDT=off  OutDataTypeStr=boolean
  Logical Operator2 : Logic  Operator=OR  AllPortsSameDT=off  OutDataTypeStr=boolean
  Logical Operator3 : Logic  Operator=NOT  AllPortsSameDT=off  OutDataTypeStr=boolean
  Logical Operator4 : Logic  Operator=OR  AllPortsSameDT=off  OutDataTypeStr=boolean
  Logical Operator5 : Logic  AllPortsSameDT=off  OutDataTypeStr=boolean
  Switch1 : Switch  Criteria=u2 > Threshold  Threshold=1  SaturateOnIntegerOverflow=off  InputSameDT=off
  Unit Delay : UnitDelay  InitialCondition=1  SampleTime=t_clock  HasFrameUpgradeWarning=on
  Q : Outport  VectorParamsAs1DForOutWhenUnconnected=off
  !Q : Outport  Port=2  VectorParamsAs1DForOutWhenUnconnected=off
  wires:
  Logical Operator/1 -> Logical Operator1/2, Logical Operator5/1
  Reset/1 -> Data Type Conversion2/1
  Constant1/1 -> Switch1/2
  Logical Operator4/1 -> Switch1/1
  Data Type Conversion1/1 -> Logical Operator2/1, Logical Operator4/1
  Switch1/1 -> Q/1, Unit Delay/1, Logical Operator3/1
  Logical Operator3/1 -> !Q/1
  Set/1 -> Data Type Conversion1/1
  Logical Operator2/1 -> Logical Operator1/1
  Unit Delay/1 -> Logical Operator2/2, Logical Operator5/2
  Logical Operator5/1 -> Logical Operator4/2
  Logical Operator1/1 -> Switch1/3
  Data Type Conversion2/1 -> Logical Operator/1

== system uz_mpc_6ph_sca/ctrl_state_machine/limited_counter ==
  limit : Inport
  enb : Inport  Port=2
  Add : Sum  Inputs=-++  AccumDataTypeStr=uint8
  Constant3 : Constant  Value=0  OutDataTypeStr=uint8  SampleTime=-1
  Constant5 : Constant  OutDataTypeStr=uint8  SampleTime=-1
  Constant6 : Constant  Value=0  OutDataTypeStr=uint8  SampleTime=-1
  Delay4 : Delay  DelayLength=1
  Relational Operator1 : RelationalOperator  OutDataTypeStr=boolean  RndMeth=Simplest  InputSameDT=off
  Switch7 : Switch  Criteria=u2 > Threshold  SaturateOnIntegerOverflow=off  InputSameDT=off
  Switch8 : Switch  Criteria=u2 > Threshold  SaturateOnIntegerOverflow=off  InputSameDT=off
  cnt : Outport
  wires:
  Constant6/1 -> Switch8/3
  Constant3/1 -> Switch7/3
  Switch8/1 -> Add/1  "trigger"
  Delay4/1 -> Add/3, Relational Operator1/1, Switch8/1
  Switch7/1 -> Add/2  "trigger"
  Constant5/1 -> Switch7/1
  Relational Operator1/1 -> Switch8/2
  Add/1 -> cnt/1, Delay4/1
  limit/1 -> Relational Operator1/2
  enb/1 -> Switch7/2

== system uz_mpc_6ph_sca/ctrl_state_machine/resetable_counter ==
  enb : Inport
  rst : Inport  Port=2
  Add : Sum  Inputs=-++  AccumDataTypeStr=uint8
  Add1 : Sum  Inputs=+-  AccumDataTypeStr=uint8
  Constant1 : Constant  Value=0  OutDataTypeStr=uint8  SampleTime=-1
  Constant3 : Constant  Value=0  OutDataTypeStr=uint8  SampleTime=-1
  Constant5 : Constant  OutDataTypeStr=uint8  SampleTime=-1
  Constant6 : Constant  Value=0  OutDataTypeStr=uint8  SampleTime=-1
  Delay4 : Delay  DelayLength=1
  Switch7 : Switch  Criteria=u2 > Threshold  SaturateOnIntegerOverflow=off  InputSameDT=off
  Switch8 : Switch  Criteria=u2 > Threshold  SaturateOnIntegerOverflow=off  InputSameDT=off
  cnt : Outport
  wires:
  Constant6/1 -> Switch8/3
  Constant3/1 -> Switch7/3
  Switch8/1 -> Add/1  "trigger"
  Switch7/1 -> Add/2  "trigger"
  Constant5/1 -> Switch7/1
  Add/1 -> cnt/1, Delay4/1
  enb/1 -> Switch7/2
  Constant1/1 -> Add1/2
  Add1/1 -> Switch8/1
  Delay4/1 -> Add/3, Add1/1
  rst/1 -> Switch8/2
